simulink model "xaui_aligner"  (Simulink 7.0)
settings: Solver=ode45  StartTime=0.0  StopTime=1e3  RelTol=1e-3
libraries: xbsIndex_r4 x32, casper_library_misc x1
settings Model: Creator=mdexter  LastModifiedBy=mdexter

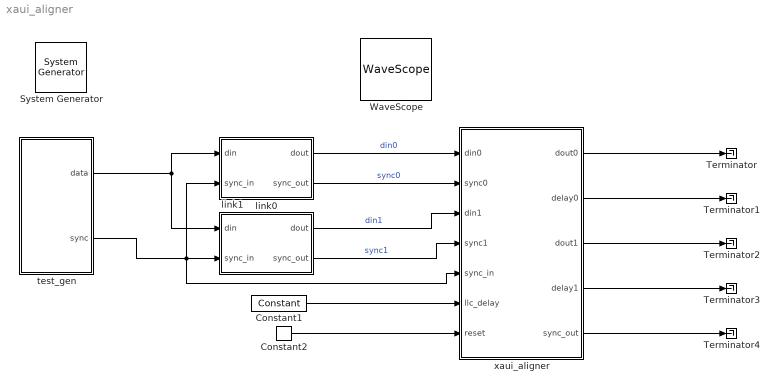
== system xaui_aligner ==
  " System Generator" : xbsIndex_r4/ System Generator  Tag=genX  SystemSampleTime=-1  xilinxfamily=Virtex4  part=xc4vsx35  speed=-10  package=ff668  synthesis_tool=XST  clock_wrapper=Clock Enables  directory=./netlist  testbench=off  simulink_period=1  sysclk_period=100  dcm_input_clock_period=100  incr_netlist=off  trim_vbits=Everywhere in SubSystem  dbl_ovrd=According to Block Masks  core_generation=According to Block Masks  run_coregen=off  deprecated_control=off  eval_field=0  block_type=sysgen
      settings: block_version=10.1.3
  Constant1 : xbsIndex_r4/Constant  arith_type=Unsigned  const=63  n_bits=16  bin_pt=0  explicit_period=on  period=1  equ=P=C  opselect=C  inp2=PCIN>>17  opr=+  inp1=P  carry=CIN  dbl_ovrd=off  block_type=constant
  Constant2 : xbsIndex_r4/Constant  arith_type=Boolean  const=0  n_bits=16  bin_pt=14  explicit_period=on  period=1  equ=P=C  opselect=C  inp2=PCIN>>17  opr=+  inp1=P  carry=CIN  dbl_ovrd=off  block_type=constant
  Terminator{,1..4} (5 alike) : Terminator
  WaveScope : xbsIndex_r4/WaveScope  block_type=wavescope
      settings: block_version=10.1.3
  link0 : Subsystem
  link1 : Subsystem
  test_gen : Subsystem
  xaui_aligner : Subsystem
  wires:
  test_gen/1(data) -> link0/1(din), link1/1(din)
  test_gen/2(sync) -> link1/2(sync_in), link0/2(sync_in), xaui_aligner/5(sync_in)
  link0/1(dout) -> xaui_aligner/1(din0)  "din0"
  link0/2(sync_out) -> xaui_aligner/2(sync0)  "sync0"
  link1/1(dout) -> xaui_aligner/3(din1)  "din1"
  link1/2(sync_out) -> xaui_aligner/4(sync1)  "sync1"
  Constant1/1 -> xaui_aligner/6(llc_delay)
  Constant2/1 -> xaui_aligner/7(reset)
  xaui_aligner/1(dout0) -> Terminator/1
  xaui_aligner/2(delay0) -> Terminator1/1
  xaui_aligner/3(dout1) -> Terminator2/1
  xaui_aligner/4(delay1) -> Terminator3/1
  xaui_aligner/5(sync_out) -> Terminator4/1

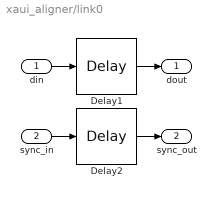
== system xaui_aligner/link0 ==
  din : Inport
  sync_in : Inport  Port=2
  Delay1 : xbsIndex_r4/Delay  en=off  latency=50  dbl_ovrd=off  reg_retiming=off  block_type=delay
  Delay2 : xbsIndex_r4/Delay  en=off  latency=50  dbl_ovrd=off  reg_retiming=off  block_type=delay
  dout : Outport
  sync_out : Outport  Port=2
  wires:
  din/1 -> Delay1/1
  Delay1/1 -> dout/1
  sync_in/1 -> Delay2/1
  Delay2/1 -> sync_out/1

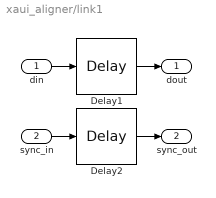
== system xaui_aligner/link1 ==
  din : Inport
  sync_in : Inport  Port=2
  Delay1 : xbsIndex_r4/Delay  en=off  latency=60  dbl_ovrd=off  reg_retiming=off  block_type=delay
  Delay2 : xbsIndex_r4/Delay  en=off  latency=60  dbl_ovrd=off  reg_retiming=off  block_type=delay
  dout : Outport
  sync_out : Outport  Port=2
  wires:
  din/1 -> Delay1/1
  Delay1/1 -> dout/1
  sync_in/1 -> Delay2/1
  Delay2/1 -> sync_out/1

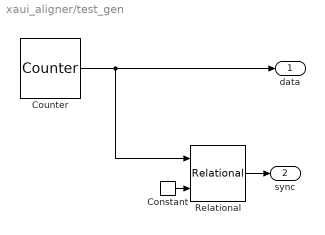
== system xaui_aligner/test_gen ==
  Constant : xbsIndex_r4/Constant  arith_type=Unsigned  const=0  n_bits=8  bin_pt=0  explicit_period=on  period=1  equ=P=C  opselect=C  inp2=PCIN>>17  opr=+  inp1=P  carry=CIN  dbl_ovrd=off  block_type=constant
  Counter : xbsIndex_r4/Counter  cnt_type=Free Running  cnt_to=Inf  operation=Up  start_count=0  cnt_by_val=1  arith_type=Unsigned  n_bits=8  bin_pt=0  load_pin=off  rst=off  en=off  explicit_period=on  period=1  dbl_ovrd=off  use_behavioral_HDL=off  use_rpm=off  implementation=Fabric  block_type=counter
  Relational : xbsIndex_r4/Relational  mode=a=b  en=off  latency=0  dbl_ovrd=off  block_type=relational
      settings: block_version=10.1.3
  data : Outport
  sync : Outport  Port=2
  wires:
  Counter/1 -> Relational/1, data/1
  Relational/1 -> sync/1
  Constant/1 -> Relational/2

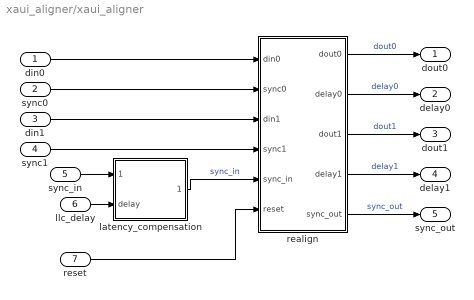
== system xaui_aligner/xaui_aligner ==
  din0 : Inport
  sync0 : Inport  Port=2
  din1 : Inport  Port=3
  sync1 : Inport  Port=4
  sync_in : Inport  Port=5
  llc_delay : Inport  Port=6
  reset : Inport  Port=7
  latency_compensation : Subsystem
  realign : Subsystem
  dout0 : Outport
  delay0 : Outport  Port=2
  dout1 : Outport  Port=3
  delay1 : Outport  Port=4
  sync_out : Outport  Port=5
  wires:
  latency_compensation/1(sync_out) -> realign/5(sync_in)  "sync_in"
  sync_in/1 -> latency_compensation/1(sync_in)
  realign/1(dout0) -> dout0/1  "dout0"
  din0/1 -> realign/1(din0)
  sync0/1 -> realign/2(sync0)
  realign/2(delay0) -> delay0/1  "delay0"
  din1/1 -> realign/3(din1)
  realign/3(dout1) -> dout1/1  "dout1"
  sync1/1 -> realign/4(sync1)
  realign/4(delay1) -> delay1/1  "delay1"
  llc_delay/1 -> latency_compensation/2(delay)
  reset/1 -> realign/6(reset)
  realign/5(sync_out) -> sync_out/1  "sync_out"

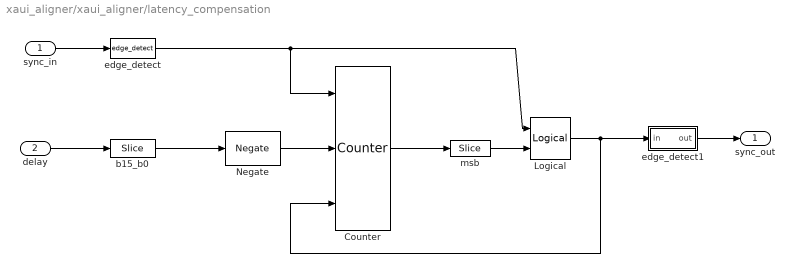
== system xaui_aligner/xaui_aligner/latency_compensation ==
  sync_in : Inport  OutDataType=sfix(16)  OutScaling=2^0
  delay : Inport  Port=2  OutDataType=sfix(16)  OutScaling=2^0
  Counter : xbsIndex_r4/Counter  cnt_type=Free Running  cnt_to=Inf  operation=Up  start_count=0  cnt_by_val=1  arith_type="Signed  (2's comp)"  n_bits=17  bin_pt=0  load_pin=on  rst=off  en=on  explicit_period=off  period=1  dbl_ovrd=off  use_behavioral_HDL=on  use_rpm=on  implementation=Fabric  block_type=counter
      settings: xl_area=[0, 0, 0, 0, 0, 0, 0]
  Logical : xbsIndex_r4/Logical  logical_function=OR  inputs=2  en=off  latency=0  precision=Full  arith_type=Unsigned  n_bits=8  bin_pt=2  align_bp=on  dbl_ovrd=off  block_type=logical
      settings: xl_area=[0, 0, 0, 0, 0, 0, 0]
  Negate : xbsIndex_r4/Negate  precision=Full  arith_type="Signed  (2's comp)"  n_bits=16  bin_pt=0  quantization=Truncate  overflow=Wrap  en=off  latency=1  dbl_ovrd=off  block_type=negate
      settings: xl_area=[0, 0, 0, 0, 0, 0, 0]  block_version=10.1.3
  b15_b0 : xbsIndex_r4/Slice  nbits=16  boolean_output=off  mode=Lower Bit Location + Width  bit1=0  base1=MSB of Input  bit0=0  base0=LSB of Input  dbl_ovrd=off  block_type=slice
      settings: infoedit="Extracts a given range of bits from each input sample and presents it at the output.  The output type is ordinarily unsigned with binary point at zero, but can be Boolean when the slice is one bit wide.<P><P>Hardware notes: In hardware this block costs nothing."  block_version=10.1.3
  edge_detect : casper_library_misc/edge_detect  SystemSampleTime=-1  edge=Rising  polarity=Active High  x_in=[0 0.08 0.08 0.16 0.16 0.24 0.24 0.32 0.32 0.4]  y_in="[-1 -1  1  1  1  1  1  1  1  1]"  x_out=[0.6 0.68 0.68 0.76 0.76 0.84 0.84 0.92 0.92 1]  y_out="[-1 -1  1  1 -1 -1 -1 -1 -1 -1]"
  edge_detect1 : Subsystem  AncestorBlock=casper_library_misc/edge_detect  mask(edge_detect){edge=Falling, polarity=Active High, x_in=[0 0.08 0.08 0.16 0.16 0.24 0.24 0.32 0.32 0.4], y_in=[1  1 -1 -1 -1 -1 -1 -1 -1 -1], x_out=[0.6 0.68 0.68 0.76 0.76 0.84 0.84 0.92 0.92 1], y_out=[-1 -1  1  1 -1 -1 -1 -1 -1 -1]}
      mask prompts: edge "Edge Type"; polarity "Output Polarity"; x_in "Input X Positions"; y_in "Input Y Positions"; x_out "Output X Positions"; y_out "Output Y Positions"
      mask help: Output is active for one-cycle after each edge of the specified type (i.e. rising, falling or both).
      mask init:
      | edge_detect_init(gcb,...
      |     'edge',edge,...
      |     'polarity',polarity,...
      |     'x_in',x_in,...
      |     'x_out',x_out,...
      |     'y_in',y_in,...
      |     'y_out',y_out);
      | 
      | x_in_num=str2num(getfield(getfield(get_param(gcb,'UserData'),'parameters'),'x_in'));
      | x_out_num=str2num(getfield(getfield(get_param(gcb,'UserData'),'parameters'),'x_out'));
      | y_in_num=str2num(getfield(getfield(get_param(gcb,'UserData'),'parameters'),'y_in'));
      | y_out_num=str2num(getfield(getfield(get_param(gcb,'UserData'),'parameters'),'y_out'));
      settings: AttributesFormatString=|
      | falling edges
      | active high
      mask Help: Output is active for one-cycle after each edge of the specified type (i.e. rising, falling, or both).  Latency is zero.
      mask StyleString: popup(Rising|Falling|Both),popup(Active High|Active Low),edit,edit,edit,edit
      mask Display:
      | plot(x_in_num,0.5+y_in_num*0.2);
      | plot(x_out_num,0.5+y_out_num*0.2);
  msb : xbsIndex_r4/Slice  nbits=1  boolean_output=on  mode=Upper Bit Location + Width  bit1=0  base1=MSB of Input  bit0=0  base0=LSB of Input  dbl_ovrd=off  block_type=slice
      settings: infoedit="Extracts a given range of bits from each input sample and presents it at the output.  The output type is ordinarily unsigned with binary point at zero, but can be Boolean when the slice is one bit wide.<P><P>Hardware notes: In hardware this block costs nothing."  block_version=10.1.3
  sync_out : Outport  OutDataType=sfix(16)  OutScaling=2^0
  wires:
  edge_detect/1 -> Counter/1, Logical/1
  sync_in/1 -> edge_detect/1
  Counter/1 -> msb/1
  msb/1 -> Logical/2
  b15_b0/1 -> Negate/1
  Negate/1 -> Counter/2
  delay/1 -> b15_b0/1
  edge_detect1/1(out) -> sync_out/1
  Logical/1 -> Counter/3, edge_detect1/1(in)

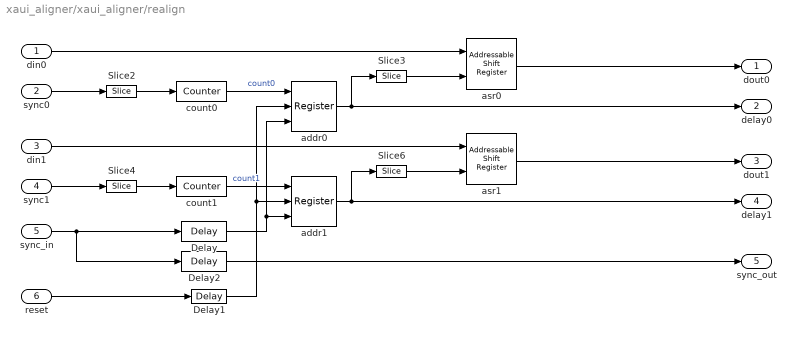
== system xaui_aligner/xaui_aligner/realign ==
  din0 : Inport  OutDataType=sfix(16)  OutScaling=2^0
  sync0 : Inport  Port=2  OutDataType=sfix(16)  OutScaling=2^0
  din1 : Inport  Port=3  OutDataType=sfix(16)  OutScaling=2^0
  sync1 : Inport  Port=4  OutDataType=sfix(16)  OutScaling=2^0
  sync_in : Inport  Port=5  OutDataType=sfix(16)  OutScaling=2^0
  reset : Inport  Port=6  OutDataType=sfix(16)  OutScaling=2^0
  Delay : xbsIndex_r4/Delay  en=off  latency=1  dbl_ovrd=off  reg_retiming=off  block_type=delay
      settings: xl_area=[1 1 0 0 0 0 0]
  Delay1 : xbsIndex_r4/Delay  en=off  latency=1  dbl_ovrd=off  reg_retiming=off  block_type=delay
      settings: xl_area=[1 1 0 0 0 0 0]
  Delay2 : xbsIndex_r4/Delay  en=off  latency=1  dbl_ovrd=off  reg_retiming=off  block_type=delay
      settings: xl_area=[1 1 0 0 0 0 0]
  Slice2 : xbsIndex_r4/Slice  nbits=1  boolean_output=on  mode=Lower Bit Location + Width  bit1=0  base1=MSB of Input  bit0=0  base0=LSB of Input  dbl_ovrd=off  block_type=slice
      settings: infoedit="Extracts a given range of bits from each input sample and presents it at the output.  The output type is ordinarily unsigned with binary point at zero, but can be Boolean when the slice is one bit wide.<P><P>Hardware notes: In hardware this block costs nothing."  block_version=10.1.3
  Slice3 : xbsIndex_r4/Slice  nbits=6  boolean_output=off  mode=Lower Bit Location + Width  bit1=0  base1=MSB of Input  bit0=0  base0=LSB of Input  dbl_ovrd=off  block_type=slice
      settings: infoedit="Extracts a given range of bits from each input sample and presents it at the output.  The output type is ordinarily unsigned with binary point at zero, but can be Boolean when the slice is one bit wide.<P><P>Hardware notes: In hardware this block costs nothing."  block_version=10.1.3
  Slice4 : xbsIndex_r4/Slice  nbits=1  boolean_output=on  mode=Lower Bit Location + Width  bit1=0  base1=MSB of Input  bit0=0  base0=LSB of Input  dbl_ovrd=off  block_type=slice
      settings: infoedit="Extracts a given range of bits from each input sample and presents it at the output.  The output type is ordinarily unsigned with binary point at zero, but can be Boolean when the slice is one bit wide.<P><P>Hardware notes: In hardware this block costs nothing."  block_version=10.1.3
  Slice6 : xbsIndex_r4/Slice  nbits=6  boolean_output=off  mode=Lower Bit Location + Width  bit1=0  base1=MSB of Input  bit0=0  base0=LSB of Input  dbl_ovrd=off  block_type=slice
      settings: infoedit="Extracts a given range of bits from each input sample and presents it at the output.  The output type is ordinarily unsigned with binary point at zero, but can be Boolean when the slice is one bit wide.<P><P>Hardware notes: In hardware this block costs nothing."  block_version=10.1.3
  addr0 : xbsIndex_r4/Register  init=hex2dec('DEC0')  rst=on  en=on  dbl_ovrd=off  block_type=register
      settings: xl_area=[3 6 0 0 0 0 0]
  addr1 : xbsIndex_r4/Register  init=hex2dec('DEC0')  rst=on  en=on  dbl_ovrd=off  block_type=register
      settings: xl_area=[3 6 0 0 0 0 0]
  asr0 : xbsIndex_r4/Addressable Shift Register  infer_latency=on  depth=64  initVector=[0]  en=off  dbl_ovrd=off  use_behavioral_HDL=off  use_rpm=on  block_type=addrsr
      settings: infoedit="Delay of configurable length.  Any element in the delay line can be addressed and driven onto the output port.<br><br>Hardware notes: Implemented using SRL16s.  If Virtex-4, Virtex-II or Spartan-3 devices are used, multiple SRLC16s are cascaded together."  xl_area=[192 0 0 384 0 0 0]  block_version=10.1.3
  asr1 : xbsIndex_r4/Addressable Shift Register  infer_latency=on  depth=64  initVector=[0]  en=off  dbl_ovrd=off  use_behavioral_HDL=off  use_rpm=on  block_type=addrsr
      settings: infoedit="Delay of configurable length.  Any element in the delay line can be addressed and driven onto the output port.<br><br>Hardware notes: Implemented using SRL16s.  If Virtex-4, Virtex-II or Spartan-3 devices are used, multiple SRLC16s are cascaded together."  xl_area=[192 0 0 384 0 0 0]  block_version=10.1.3
  count0 : xbsIndex_r4/Counter  cnt_type=Free Running  cnt_to=hex2dec('FFFF')  operation=Up  start_count=0  cnt_by_val=1  arith_type=Unsigned  n_bits=32  bin_pt=0  load_pin=off  rst=on  en=off  explicit_period=off  period=1  dbl_ovrd=off  use_behavioral_HDL=on  use_rpm=on  implementation=Fabric  block_type=counter
      settings: xl_area=[3 6 0 6 0 0 0]
  count1 : xbsIndex_r4/Counter  cnt_type=Free Running  cnt_to=hex2dec('FFFF')  operation=Up  start_count=0  cnt_by_val=1  arith_type=Unsigned  n_bits=32  bin_pt=0  load_pin=off  rst=on  en=off  explicit_period=off  period=1  dbl_ovrd=off  use_behavioral_HDL=on  use_rpm=on  implementation=Fabric  block_type=counter
      settings: xl_area=[3 6 0 6 0 0 0]
  dout0 : Outport  OutDataType=sfix(16)  OutScaling=2^0
  delay0 : Outport  Port=2  OutDataType=sfix(16)  OutScaling=2^0
  dout1 : Outport  Port=3  OutDataType=sfix(16)  OutScaling=2^0
  delay1 : Outport  Port=4  OutDataType=sfix(16)  OutScaling=2^0
  sync_out : Outport  Port=5  OutDataType=sfix(16)  OutScaling=2^0
  wires:
  count0/1 -> addr0/1  "count0"
  addr0/1 -> Slice3/1, delay0/1
  count1/1 -> addr1/1  "count1"
  addr1/1 -> Slice6/1, delay1/1
  din0/1 -> asr0/1
  asr0/1 -> dout0/1
  sync0/1 -> Slice2/1
  din1/1 -> asr1/1
  asr1/1 -> dout1/1
  sync1/1 -> Slice4/1
  sync_in/1 -> Delay/1, Delay2/1
  Slice2/1 -> count0/1
  Slice4/1 -> count1/1
  Delay/1 -> addr0/3, addr1/3
  Slice3/1 -> asr0/2
  Slice6/1 -> asr1/2
  reset/1 -> Delay1/1
  Delay1/1 -> addr0/2, addr1/2
  Delay2/1 -> sync_out/1

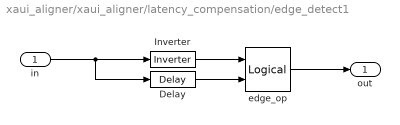
== system xaui_aligner/xaui_aligner/latency_compensation/edge_detect1 ==
  in : Inport  OutDataType=sfix(16)  OutScaling=2^0
  Delay : xbsIndex_r4/Delay  en=off  latency=1  dbl_ovrd=off  reg_retiming=off  block_type=delay
      settings: xl_area=[0, 0, 0, 0, 0, 0, 0]
  Inverter : xbsIndex_r4/Inverter  en=off  latency=0  dbl_ovrd=off  block_type=inv
      settings: xl_area=[0, 0, 0, 0, 0, 0, 0]
  edge_op : xbsIndex_r4/Logical  logical_function=AND  inputs=2  en=off  latency=0  precision=Full  arith_type=Unsigned  n_bits=8  bin_pt=2  align_bp=on  dbl_ovrd=off  block_type=logical
      settings: xl_area=[0, 0, 0, 0, 0, 0, 0]
  out : Outport  OutDataType=sfix(16)  OutScaling=2^0
  wires:
  Inverter/1 -> edge_op/1
  edge_op/1 -> out/1
  in/1 -> Inverter/1, Delay/1
  Delay/1 -> edge_op/2
